simulink model "GFLIB_Hyst_BAM_F16"  (Simulink 7.3)
settings: Solver=ode45  StartTime=0.0  StopTime=10.0  RelTol=1e-3
undefined symbols (not defined in the file): f16HystOff, f16HystOn, f16OutValOff, f16OutValOn
settings Model: Creator=B17364  LastModifiedBy=B17364

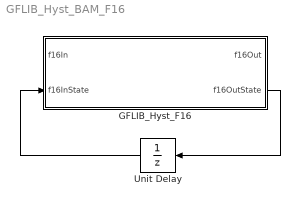
== system GFLIB_Hyst_BAM_F16 ==
  GFLIB_Hyst_F16 : Subsystem  mask(GFLIB_Hyst_F16){f16HystOn=f16HystOn, f16HystOff=f16HystOff, f16OutValOn=f16OutValOn, f16OutValOff=f16OutValOff}
      mask help: Bit accurate model of hysteresis function. All parameters as well as input and output are 16-bit integers.
      mask init:
      | pos = get_param(gcb, 'Position');width = pos(3) - pos(1); height = pos(4) - pos(2);tX=width/2;tY=height*0.9;
      mask Display: color('black');port_label('input',1,'f16In');port_label('input',2,'f16InState');port_label('output',1,'f16Out');port_label('output',2,'f16OutState');color('black');disp('GFLIB_Hyst_F16');color('blue');text(tX,tY, 'BAM', 'horizontalAlignment', 'center');
  Unit Delay : UnitDelay  SampleTime=-1
  wires:
  GFLIB_Hyst_F16/2(f16OutState) -> Unit Delay/1
  Unit Delay/1 -> GFLIB_Hyst_F16/2(f16InState)

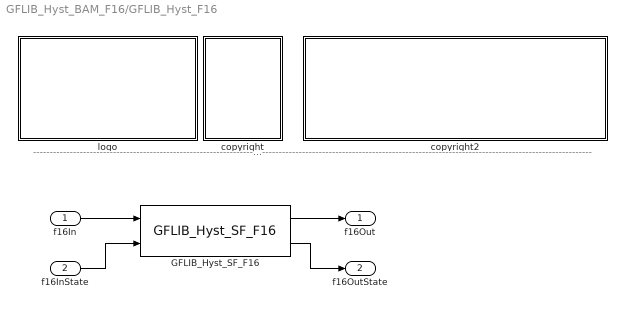
== system GFLIB_Hyst_BAM_F16/GFLIB_Hyst_F16 ==
  note: ---------------------------------------------------------------------------------------------------------------------------------------------------------------------------------------------------
  f16In : Inport  OutDataType=fixdt(1, 16)  OutScaling=2^0
  f16InState : Inport  Port=2  OutDataType=fixdt(1, 16)  OutScaling=2^0
  GFLIB_Hyst_SF_F16 : S-Function  FunctionName=GFLIB_Hyst_SF_F16  Parameters=f16HystOn,f16HystOff,f16OutValOn,f16OutValOff  EnableBusSupport=off
  copyright : Subsystem
      mask Display: text(10,90,'FILE:');text(10,75,'DESRIPTION:')text(10,60,'COPYRIGHT:')text(10,45,'VERSION:')text(10,30,'DATE:')
  copyright2 : Subsystem
      mask Display: text(10,90,'GFLIB_Hyst_BAM_F16.mdl');text(10,75,'Hysteresis function.');text(10,60,'Freescale')text(10,45,'0.1');text(10,30,'09-Apr-2014');
  logo : Subsystem
      mask Display: image(imread('logo.jpg'))
  f16Out : Outport  OutDataType=fixdt(1, 16)  OutScaling=2^0
  f16OutState : Outport  Port=2  OutDataType=fixdt(1, 16)  OutScaling=2^0
  wires:
  f16In/1 -> GFLIB_Hyst_SF_F16/1
  GFLIB_Hyst_SF_F16/1 -> f16Out/1
  GFLIB_Hyst_SF_F16/2 -> f16OutState/1
  f16InState/1 -> GFLIB_Hyst_SF_F16/2

== system GFLIB_Hyst_BAM_F16/GFLIB_Hyst_F16/copyright ==

== system GFLIB_Hyst_BAM_F16/GFLIB_Hyst_F16/copyright2 ==

== system GFLIB_Hyst_BAM_F16/GFLIB_Hyst_F16/logo ==
